simulink model "simulationSprint2"  (R2018b)
settings: Solver=FixedStepAuto  StartTime=0.0  StopTime=10  FixedStep=0.01  MaxStep=100e-3  RelTol=1e-3
(part 3 of 3)

== stateflow chart simulationSprint2/Req22 ==
  note: The module responsible by test the requeriment nine.
      |
      | Notice : i_ means input signals
      | o_ means output signals
      |
      | Input :
      | i_enable - Start the test. 1- Start test . 0 - Do nothing.
      | i_desiredTest - Test Number Value. All the modules recieve the
      | signal and decide either execute the test. Ex: Value "1" means that will being testing the requeriment 1.
      | i_MotorState. 1 - On ; 0 - Off .
      | i_headLampPark. 1 - Lamp On ; 0 - Lamp Off.
      | i_OverHeadLamp - State the Head Lamp. 1 - Light On ; 0 - Light Off.
      | i_RearLamps. 1 - Light On ; 0 - Light Off .
      | i_battery. Level of battery. Range 0 - 100 %. Note. Using olny here to simulation an especified battery value. other test, battery value is get directly on the BMS module.
      |
      | Output :
      | o_TestResult - Result of test. 1 - Test ran correctly ; 2 - Test ran incorrectly.
      | o_TestDone - Test has been completed. 1 - Completed ;
      | o_keyfob - Signal that indicates if the key is inside or not from the car. 1 - Key inside ; 0 - Key outside.
      | o_keyCommand - Signal to lock or unlock the car. "1 - lock the car ; 2 - Unlock the car" ; 0 - Do nothing.
      | o_startButtom - Signal to start or off the car. 1- Car Start ; 0 - Car off.
      | o_gear = gear State ; 1 - Park ; 0 - Engaged.
      | o_doorAction - Action in the door . 1 - Opening door 0 - Closing Door
      | o_brake = Car Brake pedal. Range 0 - 100 .
      | o_battery. Level Battery . Range 0 - 100 %. Note. Using olny here to simulation an especified battery value. other test, battery value is get directly on the BMS module.
      | o_headLamp - Light mode.
  state state_putKeyIntothecar
    during :
    o_keyfobcommand = 2 ;
    on after(200,msec):
    o_keyfobcommand = 0 ;
    on after(400,msec):
    o_keyfob = 1;
    o_gear = 1 ;
    on after(600,msec):
  state state_setbattery
    o_battery = 1 ;
    on after(200, msec):
    o_DoorAction = 1 ;
    o_HeadLamp = 1 ;
    o_brake = 1;
    exit :
    o_DoorAction = 0 ;
    o_HeadLamp = 0 ;
    o_brake = 0;
  state state_idle
    exit :
    r_aux = 0 ;
    o_keyfobcommand = 0;
    o_keyfob =0;
    o_gear = 1;
  state State_error
    entry :
    during:
    o_TestResult =0;
    o_testDone =1 ;
    on after(200,msec):
    r_aux =1;
    exit :
    r_aux =0;
  state turnOncar
    during :
    o_startButtom
  state testeWithCarOn
    during :
    o_DoorAction = 1 ;
    o_HeadLamp = 1 ;
    o_brake = 2;
  state State_feat_ok
    entry :
    during:
    o_TestResult =1;
    o_testDone =1;
    o_startButtom=0;
    on after(200,msec):
    r_aux =1;
    exit:
    r_aux =0;
  state state_update
    entry:
    r_aux = 0;
    during:
    on after(1,sec):
    o_TestResult =0;
    o_testDone = 0;
    r_aux =1 ;
    exit:
  state_putKeyIntothecar -> state_setbattery : after(1,sec)
  (default) -> state_idle
  state_idle -> state_putKeyIntothecar : [i_enable==1 && i_desiredTest == 22 ]
  state_update -> state_idle : [r_aux ==1]
  state_setbattery -> State_error [order 2] : [after(3,sec) && (i_battery ~= 70 || i_headLampPark~=0 || i_OverHeadLamp ~=0 || i_RearLamp ~=0)]
  state_setbattery -> turnOncar [order 1] : [after(3,sec) && i_battery == 70 && i_headLampPark==0 && i_OverHeadLamp ==0 && i_RearLamp ==0]
  turnOncar -> testeWithCarOn [order 2] : [i_motorState == 1 && after(1,sec)]
  turnOncar -> State_error [order 1] : [i_motorState == 0 && after(1,sec)]
  testeWithCarOn -> State_error [order 2] : [after(3,sec) && (i_battery ~= 70 || i_headLampPark~=0 || i_OverHeadLamp ~=0 || i_RearLamp ~=0)]
  testeWithCarOn -> State_feat_ok [order 1] : [after(3,sec) && i_battery == 70 && i_headLampPark==0 && i_OverHeadLamp ==0 && i_RearLamp ==0]
  State_error -> state_update : [r_aux==1]
  State_feat_ok -> state_update : [r_aux==1]
  data: i_enable input size=1; i_desiredTest input int8 size=1; o_TestResult output int8 size=1; o_testDone output int8 size=1; r_aux local; i_motorState input int8 size=1; o_gear output int8 size=1; o_keyfob output int8 size=1; o_keyfobcommand output int8 size=1; o_startButtom output int8 size=1; o_DoorAction output; i_headLampPark input; i_OverHeadLamp input; i_RearLamp input; i_battery input; o_battery output; o_HeadLamp output; o_brake output

== stateflow chart simulationSprint2/Req23 ==
  note: The module responsible by test the requeriment nine.
      |
      | Notice : i_ means input signals
      | 		o_ means output signals
      |
      | Input :
      | i_enable - Start the test. 1- Start test . 0 - Do nothing.
      | i_desiredTest - Test Number Value. All the modules recieve the
      | signal and decide either execute the test. Ex: Value "1" means that will being testing the requeriment 1.
      | i_CarLockState. 1 - Car unlock ; 0 - Car Lock.
      |
      |
      | Output :
      | o_TestResult - Result of test. 1 - Test ran correctly ; 2 - Test ran incorrectly.
      | o_TestDone - Test has been completed. 1 - Completed ;
      | o_keyfobCode -  Key Code to send together the unlock key signal . 60 and 70 are valid code, any other is invalid code.
      | o_keyCommand - Signal to lock or unlock the car. "1 - lock the car ; 2 - Unlock the car" ;  0 - Do nothing.
  state state_putKeyIntheCar3
    during :
    o_keyfobCode = 60;
    on after(50,msec):
    o_keyfobcommand =1;
    on after(100,msec):
    o_keyfobcommand =0;
  state state_idle
    entry :
    r_aux = 0 ;
    o_keyfobcommand = 0;
  state state_putKeyIntheCar
    during :
    o_keyfobCode = 65;
    on after(50,msec):
    o_keyfobcommand =2;
    on after(100,msec):
    o_keyfobcommand =0;
  state state_putKeyIntheCar1
    during :
    o_keyfobCode = 60;
    on after(50,msec):
    o_keyfobcommand =2;
    on after(100,msec):
    o_keyfobcommand =0;
  state State_error
    entry :
    during:
    o_TestResult =0;
    o_testDone =1 ;
    on after(200,msec):
    r_aux =1;
    exit :
    r_aux =0;
  state state_putKeyIntheCar2
    during :
    o_keyfobCode = 70;
    on after(50,msec):
    o_keyfobcommand =1;
    on after(100,msec):
    o_keyfobcommand =0;
  state state_update
    entry:
    r_aux = 0;
    during:
    on after(1,sec):
    o_TestResult =0;
    o_testDone = 0;
    r_aux =1 ;
    exit:
  state State_feat_ok
    during:
    o_TestResult =1;
    o_testDone =1;
    on after(100,msec):
    r_aux =1;
    exit:
    r_aux =0;
  state_idle -> state_putKeyIntheCar3 : [i_enable==1 && i_desiredTest == 23 ]
  (default) -> state_idle
  state_putKeyIntheCar3 -> state_putKeyIntheCar [order 1] : [after(500,msec) && i_CarLockStatus == 0 ]
  state_putKeyIntheCar3 -> State_error [order 2] : [after(500,msec)  && i_CarLockStatus ~=0 ]
  state_putKeyIntheCar -> state_putKeyIntheCar1 [order 2] : [after(500,msec) && i_CarLockStatus == 0 ]
  state_update -> state_idle : [r_aux ==1]
  state_putKeyIntheCar1 -> State_error [order 2] : [after(500,msec) && i_CarLockStatus ~= 1 ]
  state_putKeyIntheCar1 -> state_putKeyIntheCar2 [order 1] : [after(500,msec) &&  i_CarLockStatus == 1 ]
  state_putKeyIntheCar -> State_error [order 1] : [after(500,msec)  && i_CarLockStatus ~=0 ]
  state_putKeyIntheCar2 -> State_error [order 1] : [after(500,msec) && i_CarLockStatus ~= 0 ]
  state_putKeyIntheCar2 -> State_feat_ok [order 2] : [after(500,msec) && i_CarLockStatus == 0 ]
  State_error -> state_update : [r_aux==1]
  State_feat_ok -> state_update : [r_aux==1]
  data: i_enable input size=1; i_desiredTest input int8 size=1; o_TestResult output int8 size=1; o_testDone output int8 size=1; r_aux local; o_keyfobcommand output int8 size=1; o_keyfobCode output; i_CarLockStatus input

== stateflow chart simulationSprint2/Req24 ==
  note: The module responsible by test the requeriment nine.
      |
      | Notice : i_ means input signals
      | 		o_ means output signals
      |
      | Input :
      | i_enable - Start the test. 1- Start test . 0 - Do nothing.
      | i_desiredTest - Test Number Value. All the modules recieve the
      | signal and decide either execute the test. Ex: Value "1" means that will being testing the requeriment 1.
      | i_hoodState. Status of the Hood.  1 - Open ; 0 - Close .
      | i_trunkState. Status of the Trunk.  1 - Open ; 0 - Close .
      | i_CarLockStatus. Car Lock Status - 1 - Car unlock ; 0 - Car Lock.
      |
      | Output :
      | o_TestResult - Result of test. 1 - Test ran correctly ; 2 - Test ran incorrectly.
      | o_TestDone - Test has been completed. 1 - Completed ;
      | o_keyCommand - Signal to lock or unlock the car. "1 - lock the car ; 2 - Unlock the car" ;  0 - Do nothing.
      | o_keyfobCode -  Key Code to send together the unlock key signal . 60 and 70 are valid code, any other is invalid code.
      | o_trunkState - Output to simulate the trunk state - 1 - Open ; 0 - Close.
      | o_hoodState - Output to simulate the hood state - 1 - Open ; 0 - Close.
      | o_keyfob - Signal that indicates if the key is inside or not from the car. 1 - Key inside ; 0 - Key outside ; 2 - Key Near.
  state state_idle
    entry :
    r_aux = 0 ;
    o_keyfobcommand = 0;
    o_keyfob = 0;
  state stateTest
    entry :
    o_hoodState = 1 ;
    o_trunkState = 1 ;
    exit :
    o_hoodState = 0 ;
    o_trunkState = 0 ;
  state state_putKeyIntheCar
    during :
    o_keyfobCode = 60;
    on after(50,msec):
    o_keyfobcommand =2;
    on after(100,msec):
    o_keyfobcommand =0;
    exit :
    o_keyfob = 2;
  state stateTestWithCarOn
    entry :
    o_hoodState = 1 ;
    o_trunkState = 1 ;
  state State_error
    entry :
    during:
    o_TestResult =0;
    o_testDone =1 ;
    on after(200,msec):
    r_aux =1;
    exit :
    r_aux =0;
  state State_feat_ok
    during:
    o_TestResult =1;
    o_testDone =1;
    on after(100,msec):
    r_aux =1;
    exit:
    r_aux =0;
  state state_update
    entry:
    r_aux = 0;
    during:
    on after(1,sec):
    o_TestResult =0;
    o_testDone = 0;
    r_aux =1 ;
    exit:
  (default) -> state_idle
  stateTest -> state_putKeyIntheCar [order 1] : [after(200,msec) && i_trunkState == 0 && i_hoodState==0]
  state_idle -> stateTest : [i_enable==1 && i_desiredTest == 24 ]
  state_update -> state_idle : [r_aux ==1]
  stateTestWithCarOn -> State_feat_ok [order 2] : [after(200,msec) && i_trunkState == 1 && i_hoodState==1]
  state_putKeyIntheCar -> stateTestWithCarOn [order 1] : [after(500,msec) && i_CarLockStatus == 1 ]
  stateTest -> State_error [order 2] : [i_trunkState == 0 && i_hoodState==0 && after(200,msec)]
  state_putKeyIntheCar -> State_error [order 2] : [after(500,msec)  && i_CarLockStatus ~=1 ]
  stateTestWithCarOn -> State_error [order 1] : [after(200,msec) && i_trunkState == 0 && i_hoodState==0]
  State_error -> state_update : [r_aux==1]
  State_feat_ok -> state_update : [r_aux==1]
  data: i_enable input size=1; i_desiredTest input int8 size=1; o_TestResult output int8 size=1; o_testDone output int8 size=1; r_aux local; o_keyfobcommand output int8 size=1; o_keyfobCode output; i_hoodState input; o_trunkState output; o_hoodState output; i_trunkState input; i_CarLockStatus input; o_keyfob output

== stateflow chart simulationSprint2/Req25 ==
  note: The module responsible by test the requeriment nine.
      |
      | Notice : i_ means input signals
      | 		o_ means output signals
      |
      | Input :
      | i_enable - Start the test. 1- Start test . 0 - Do nothing.
      | i_desiredTest - Test Number Value. All the modules recieve the
      | signal and decide either execute the test. Ex: Value "1" means that will being testing the requeriment 1.
      | i_hasCode = Key Code recorded in the modules . 60 and 70 are valid code, any other is invalid code.
      | i_CarLockState. 1 - Car unlock ; 0 - Car Lock.
      |
      |
      | Output :
      | o_TestResult - Result of test. 1 - Test ran correctly ; 2 - Test ran incorrectly.
      | o_TestDone - Test has been completed. 1 - Completed ;
      | o_keyfobCode -  Key Code to send together the unlock key signal . 60 and 70 are valid code, any other is invalid code.
      | o_keyCommand - Signal to lock or unlock the car. "1 - lock the car ; 2 - Unlock the car" ;  0 - Do nothing.
  state state_putKeyIntheCar1
    during :
    o_keyfobCode = 5;
    on after(10,msec):
    o_keyfobCode = 1;
    on after(20,msec):
    o_keyfobCode = 1;
    on after(30,msec):
    o_keyfobCode = 1;
    on after(40,msec):
    o_keyfobCode = 2;
    on after(50,msec):
    o_keyfobCode = 3;
  state state_idle
    entry :
    r_aux = 0 ;
    o_keyfobCode = 0;
  state State_error
    entry :
    during:
    o_TestResult =0;
    o_testDone =1 ;
    on after(200,msec):
    r_aux =1;
    exit :
    r_aux =0;
  state state_update
    entry:
    r_aux = 0;
    during:
    on after(1,sec):
    o_TestResult =0;
    o_testDone = 0;
    r_aux =1 ;
    exit:
  state State_feat_ok
    during:
    o_TestResult =1;
    o_testDone =1;
    on after(100,msec):
    r_aux =1;
    exit:
    r_aux =0;
  (default) -> state_idle
  state_idle -> state_putKeyIntheCar1 : [i_enable==1 && i_desiredTest == 25 ]
  state_update -> state_idle : [r_aux ==1]
  state_putKeyIntheCar1 -> State_error [order 2] : [after(500,msec)  && i_CarLockStatus ~= 1 ]
  state_putKeyIntheCar1 -> State_feat_ok [order 1] : [after(1.5,sec) && i_CarLockStatus == 1 ]
  State_error -> state_update : [r_aux==1]
  State_feat_ok -> state_update : [r_aux==1]
  data: i_enable input size=1; i_desiredTest input int8 size=1; o_TestResult output int8 size=1; o_testDone output int8 size=1; r_aux local; o_keyfobCode output; i_CarLockStatus input

== stateflow chart simulationSprint2/Req26 ==
  note: The module responsible by test the requeriment nine.
      |
      | Notice : i_ means input signals
      | 		o_ means output signals
      |
      | Input :
      | i_enable - Start the test. 1- Start test . 0 - Do nothing.
      | i_desiredTest - Test Number Value. All the modules recieve the
      | signal and decide either execute the test. Ex: Value "1" means that will being testing the requeriment 1.
      | i_CarLockState. 1 - Car unlock ; 0 - Car Lock.
      | i_distance = kilometers that the car can walk until the end of the gasoline in the tank.
      | i_gasolineQty = Amount of gasoline.
      |
      |
      | Output :
      | o_TestResult - Result of test. 1 - Test ran correctly ; 2 - Test ran incorrectly.
      | o_TestDone - Test has been completed. 1 - Completed ;
      | o_keyfobCode -  Key Code to send together the unlock key signal . 60 and 70 are valid code, any other is invalid code.
      | o_keyCommand - Signal to lock or unlock the car. "1 - lock the car ; 2 - Unlock the car" ;  0 - Do nothing.
  state state_idle
    entry :
    r_aux = 0 ;
    o_keyfobcommand = 0;
  state state_putKeyIntheCar1
    during :
    o_keyfobCode = 60;
    on after(50,msec):
    o_keyfobcommand =2;
    on after(50,msec):
    o_keyfobcommand =0;
  state State_error
    entry :
    during:
    o_TestResult =0;
    o_testDone =1 ;
    on after(200,msec):
    r_aux =1;
    exit :
    r_aux =0;
  state state_update
    entry:
    r_aux = 0;
    during:
    on after(1,sec):
    o_TestResult =0;
    o_testDone = 0;
    r_aux =1 ;
    exit:
  state State_feat_ok
    during:
    o_TestResult =1;
    o_testDone =1;
    on after(100,msec):
    r_aux =1;
    exit:
    r_aux =0;
  (default) -> state_idle
  state_idle -> state_putKeyIntheCar1 : [i_enable==1 && i_desiredTest == 25 ]
  state_putKeyIntheCar1 -> State_error [order 2] : [after(500,msec)  && i_CarLockStatus ~= 0 ]
  state_update -> state_idle : [r_aux ==1]
  state_putKeyIntheCar1 -> (junction 98) [order 1] : [after(500,msec) && i_CarLockStatus == 0 ]
  (junction 98) -> State_error [order 2] : [i_distance ~=i_gasolineQty * YieldCar]
  (junction 98) -> State_feat_ok [order 1] : [i_distance ==i_gasolineQty * YieldCar]
  State_error -> state_update : [r_aux==1]
  State_feat_ok -> state_update : [r_aux==1]
  data: i_enable input size=1; i_desiredTest input int8 size=1; o_TestResult output int8 size=1; o_testDone output int8 size=1; r_aux local; o_keyfobcommand output int8 size=1; o_keyfobCode output; i_CarLockStatus input; i_distance input; i_gasolineQty input; YieldCar local =15000

== stateflow chart simulationSprint2/Chart2 ==
  state state_idle
    during :
    if (i_codeKey == 70)
    o_keyValue1 = 1 ;
    o_keyValue2 = 0 ;
    o_keyValue3 = 0 ;
    elseif (i_codeKey == 60)
    o_keyValue1 = 0 ;
    o_keyValue2 = 1 ;
    o_keyValue3 = 0 ;
    else
    o_keyValue1 = 0 ;
    o_keyValue2 = 0 ;
    o_keyValue3 = 1 ;
    end
  (default) -> state_idle
  data: i_codeKey input; o_keyValue1 output; o_keyValue2 output; o_keyValue3 output
